simulink model "Vorlage_Gesamtanlage_JaehoCHa"  (R2022a)
settings: Solver=ode3  StartTime=0.0  StopTime=200  FixedStep=0.01  MaxStep=1  MinStep=0.005  RelTol=1e-3  AbsTol=10  EnableMultiTasking=on
values from neighbouring files (symbols this model uses):
  A = 5    [Parameter.m]
  Flaschengroesse = 10    [Parameter.m]
  I = 0.5    [Parameter.m]
  igetr = 1080    [Parameter.m]
  K = 8    [Parameter.m]
  MaxFlaschen = 25    [Parameter.m]
  MRK = 1    [Parameter.m]
  numA = 0    [Parameter.m]
  PassSilo1 = 1    [Parameter.m]
  PassSilo2 = 1    [Parameter.m]
  PHI = 0.001    [Parameter.m]
  Ra = 40    [Parameter.m]
  SizeSilo1 = 15    [Parameter.m]
  SizeSilo2 = 15    [Parameter.m]
  U = 24    [Parameter.m]
  v_band_abfuhr_set = 2    [Parameter.m]
  v_band_arbeit_set = 30    [Parameter.m]
  v_band_zufuhr_set = 10    [Parameter.m]
  v_umsetzer_greifer_set = 400    [Parameter.m]
  v_umsetzer_set = 80    [Parameter.m]
  v_ve1_set = 400    [Parameter.m]
  v_ve2_set = 400    [Parameter.m]
undefined symbols (not defined in the file or in its folder): Limits
libraries: simulink x94
(part 3 of 3)

== system Vorlage_Gesamtanlage_JaehoCHa/Abfüllanlage/Flaschen_data/Flaschenstarter/in_Flaschenzähler ==
  Signal : Inport
  Constant : Constant
  Constant1 : Constant  Value=0
  Logical Operator : Logic  AllPortsSameDT=off
  Memory : Memory
  Memory1 : Memory
  Relational Operator : RelationalOperator  Operator===  InputSameDT=off
  Relational Operator1 : RelationalOperator  Operator===  InputSameDT=off
  Sum : Sum  Inputs=|++  OutDataTypeStr=uint16  SaturateOnIntegerOverflow=on
  Rising Edge : Outport
  Count : Outport  Port=2
  wires:
  Signal/1 -> Memory/1, Relational Operator/2
  Constant/1 -> Relational Operator/1
  Relational Operator/1 -> Logical Operator/1
  Constant1/1 -> Relational Operator1/2
  Memory/1 -> Relational Operator1/1
  Relational Operator1/1 -> Logical Operator/2
  Logical Operator/1 -> Sum/1, Rising Edge/1
  Memory1/1 -> Sum/2
  Sum/1 -> Count/1, Memory1/1

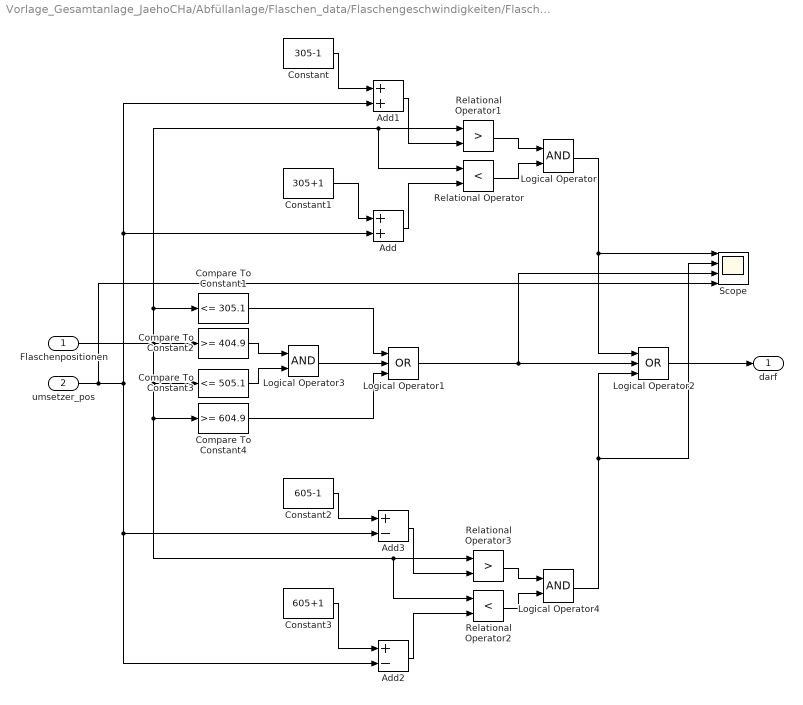
== system Vorlage_Gesamtanlage_JaehoCHa/Abfüllanlage/Flaschen_data/Flaschengeschwindigkeiten/Flaschenabstandsüberwachung/Umsetzer darf mitnehmen ==
  Flaschenpositionen : Inport
  umsetzer_pos : Inport  Port=2
  Add : Sum
  Add1 : Sum
  Add2 : Sum  Inputs=+-
  Add3 : Sum  Inputs=+-
  Compare To Constant1 : simulink/Logic and Bit Operations/Compare To Constant  relop=<=  const=305.1  OutDataTypeStr=uint8  ZeroCross=off
  Compare To Constant2 : simulink/Logic and Bit Operations/Compare To Constant  relop=>=  const=404.9  OutDataTypeStr=uint8  ZeroCross=off
  Compare To Constant3 : simulink/Logic and Bit Operations/Compare To Constant  relop=<=  const=505.1  OutDataTypeStr=uint8  ZeroCross=off
  Compare To Constant4 : simulink/Logic and Bit Operations/Compare To Constant  relop=>=  const=604.9  OutDataTypeStr=uint8  ZeroCross=off
  Constant : Constant  Value=305-1
  Constant1 : Constant  Value=305+1
  Constant2 : Constant  Value=605-1
  Constant3 : Constant  Value=605+1
  Logical Operator : Logic  AllPortsSameDT=off  OutDataTypeStr=boolean
  Logical Operator1 : Logic  Operator=OR  Inputs=3  AllPortsSameDT=off  OutDataTypeStr=boolean
  Logical Operator2 : Logic  Operator=OR  Inputs=3  AllPortsSameDT=off  OutDataTypeStr=boolean
  Logical Operator3 : Logic  AllPortsSameDT=off  OutDataTypeStr=boolean
  Logical Operator4 : Logic  AllPortsSameDT=off  OutDataTypeStr=boolean
  Relational Operator : RelationalOperator  Operator=<  OutDataTypeStr=boolean  InputSameDT=off
  Relational Operator1 : RelationalOperator  Operator=>  OutDataTypeStr=boolean  InputSameDT=off
  Relational Operator2 : RelationalOperator  Operator=<  OutDataTypeStr=boolean  InputSameDT=off
  Relational Operator3 : RelationalOperator  Operator=>  OutDataTypeStr=boolean  InputSameDT=off
  Scope : Scope  NumInputPorts=4
  darf : Outport
  wires:
  Logical Operator2/1 -> darf/1
  Logical Operator1/1 -> Logical Operator2/2, Scope/3
  Compare To Constant1/1 -> Logical Operator1/1
  Logical Operator/1 -> Logical Operator2/1, Scope/1
  Constant/1 -> Add1/1
  Add1/1 -> Relational Operator1/2
  Relational Operator1/1 -> Logical Operator/1
  Relational Operator/1 -> Logical Operator/2
  Add/1 -> Relational Operator/2
  Constant1/1 -> Add/1
  Compare To Constant2/1 -> Logical Operator3/1
  Compare To Constant3/1 -> Logical Operator3/2
  Logical Operator3/1 -> Logical Operator1/2
  Compare To Constant4/1 -> Logical Operator1/3
  Logical Operator4/1 -> Logical Operator2/3, Scope/2
  Constant2/1 -> Add3/1
  Add3/1 -> Relational Operator3/2
  Relational Operator3/1 -> Logical Operator4/1
  Relational Operator2/1 -> Logical Operator4/2
  Add2/1 -> Relational Operator2/2
  Constant3/1 -> Add2/1
  umsetzer_pos/1 -> Add2/2, Add3/2, Add/2, Add1/2, Scope/4
  Flaschenpositionen/1 -> Compare To Constant2/1, Compare To Constant3/1, Compare To Constant4/1, Relational Operator3/1, Relational Operator2/1, Compare To Constant1/1, Relational Operator1/1, Relational Operator/1

== stateflow chart Vorlage_Gesamtanlage_JaehoCHa/Abfüllanlage/Drehscheibe/Sensor ==
  state Start
    en: beep = 0;
  state Beep
    en: beep=1;
  (default) -> Start
  Start -> Beep : [ml.mod(winkel, 90) <=2 | ml.mod(winkel, 90) >=88]
  Beep -> Start : [ml.mod(winkel, 90) >2 && ml.mod(winkel, 90) <88]
  data: winkel input double; beep output boolean

== stateflow chart Vorlage_Gesamtanlage_JaehoCHa/Abfüllanlage/Fehlererkennung/Volle Flasche zum Teller zurück/Chart ==
  state Greife_Flasche_Teller
    entry: error = 0;
  state Oeffne_Greifer_Band
  state Warte_auf_VE2
  state Volle_Flasche_gegriffen
  state Greifer_gestartet
    entry: error = 1;
  state Flasche_weg
  (default) -> Greife_Flasche_Teller
  Flasche_weg -> Greife_Flasche_Teller
  Greife_Flasche_Teller -> Oeffne_Greifer_Band : [I_teller_behaelter_hinten == 1 && i_greifer_zu == 1 && i_umsetz_teller == 1]
  Oeffne_Greifer_Band -> Warte_auf_VE2 : [i_greifer_auf == 1 && i_umsetz_band == 1]
  Volle_Flasche_gegriffen -> Greifer_gestartet [order 1] : [o_umsetz_teller==1]
  Warte_auf_VE2 -> Volle_Flasche_gegriffen [order 2] : [i_greifer_zu == 1]
  Warte_auf_VE2 -> Flasche_weg [order 1] : [i_ve2_herein == 1]
  Volle_Flasche_gegriffen -> Flasche_weg [order 2] : after(5,sec)
  data: I_teller_behaelter_hinten input; i_greifer_zu input; i_umsetz_teller input; i_greifer_auf input; i_umsetz_band input; i_ve2_herein input; error output; o_umsetz_teller input

== stateflow chart Vorlage_Gesamtanlage_JaehoCHa/Steuerung ==
  state Intelligenz [parallel]
    settings: executionOrder=6
    state Anfangszustand
    state Baender_an
      en:send(e_baender_an,Baender);
    state Umsetzer_zu_band
      en:send(e_umsetzer_zu_band,Umsetzer);
      %Bedingung
      %Greifer auf
      %Bedingung nach Fullen
      %Greifer zu
    state Vereinzeler1_open
      en:send(e_ve1_open,VE1_2);
      %Bedingungen
      %Umsetzer auf Band, Greifer ist auf
      %Drehteller ist leer auf der Position
      %keine Flasche an Vereinzeler2
    state Umsetzer_zu_teller
      en:send(e_umsetzer_zu_teller,Umsetzer);
      %Bedingung
      %Greifer zu
    state Greifer_leer_Flasche
      en:send(e_greifer_zu,Umsetzer);
      %Bedingung
      %ve1 offnen
      %eine Flasche an Vereinzeler2
    state Drehteller_ausgerichtet
      en:send(e_Teller_ausgerichtet,Teller);
      %Bedingung
      %Teller ausgerichtet
    state Drehteller_drehen
      en:send(e_Teller_drehen,Teller);
      %Bedingung
      %Greifer open
      % Beidingung nach dem Fulllen
      %warten 2sec
    state Greifer_leer_flasche_los
      en:send(e_greifer_auf,Umsetzer);
      %Bedingung
      %Umsetzer auf Teller
    state Silos_open
      en:send(e_silos_open,Silos);
    state Silos_close
      en:send(e_silos_close,Silos);
    state Greifer_befuellte_Flasche
      en:send(e_greifer_zu,Umsetzer);
    state Umsetzer_zu_band1
      en:send(e_umsetzer_zu_band,Umsetzer);
    state Greifer_befuellte_Flasche_los
      en:send(e_greifer_auf,Umsetzer);
    state Vereinzeler2_open
      en:send(e_ve2_open,VE1_2)
    (default) -> Anfangszustand
    Anfangszustand -> Baender_an
    Baender_an -> Umsetzer_zu_band : [i_umsetzer[3] == 1]
    Greifer_leer_Flasche -> Umsetzer_zu_teller : [i_umsetzer[4] == 1]
    Umsetzer_zu_band -> Vereinzeler1_open : [i_umsetzer[1] == 1 &&i_umsetzer[3]==1&& i_vereinzeler[5] == 1 && i_vereinzeler[6]==0 && i_teller[2]==0]
    Vereinzeler2_open -> Umsetzer_zu_teller [order 2] : [i_silo[2]==1 && i_vereinzeler[5]==0]
    Vereinzeler1_open -> Greifer_leer_Flasche : [ i_vereinzeler[6] == 1]%check
    Silos_close -> Umsetzer_zu_band [order 2] : after(2,sec)[i_teller[2] ==0]%falls keine Flasche auf Teller behaelter
    Drehteller_ausgerichtet -> Umsetzer_zu_band [order 2] : [i_silo[2] == 0 && i_teller[2] ==0]%falls keine Flasche unter Silo und auf Tellerbehaelter
    Umsetzer_zu_teller -> Greifer_leer_flasche_los : [i_umsetzer[2]==1]
    Vereinzeler2_open -> Vereinzeler1_open [order 1] : [i_vereinzeler[4] == 1 && i_vereinzeler[5]==1]%flasche schieben
    Greifer_leer_flasche_los -> Drehteller_drehen : after(2,sec)[i_umsetzer[3]==1]
    Drehteller_drehen -> Drehteller_ausgerichtet : after(0.5,sec)[i_teller[1] == 1]
    Drehteller_ausgerichtet -> Silos_open [order 1] : [i_silo[2]==1 &&(i_silo[3] == 0&&i_silo[4]==0) ] %falls eine Flasche unter teller und beide Silo voll
    Silos_open -> Silos_close : [i_silo[1] == 0]% Flasche unter Silo und voll
    Silos_close -> Greifer_befuellte_Flasche [order 1] : after(2,sec)[i_teller[2]==1]
    Umsetzer_zu_band1 -> Greifer_befuellte_Flasche_los : [i_umsetzer[1]==1]
    Greifer_befuellte_Flasche_los -> Vereinzeler2_open : [i_umsetzer[3]==1&&i_vereinzeler[6]==1]
    Greifer_befuellte_Flasche -> Umsetzer_zu_band1 : [i_umsetzer[4]==1]
  state Umsetzer [parallel]
    settings: executionOrder=1
    state Anfangszustand_Umsetzer
      %umsetzer Band(1), teller(2)
      en:o_umsetzer[1] = 0;
      en:o_umsetzer[2] = 0;
      %Greifer auf(3), zu(4)
      en:o_umsetzer[3] = 1;
      en:o_umsetzer[4] = 0;
      %Umsetzer in Richtung Teller
      %Greifer zu
      %unbenutzte Aktoren soll ausgeschaltet sein.
      %Frage: ist Anfangszustand im Programm schon gegeben ?
    state Bandzustand_Umsetzer
      %umsetzer Band(1), teller(2)
      en:o_umsetzer[1] = 1;
      en:o_umsetzer[2] = 0;
      %Greifer auf(3), zu(4)
      en:o_umsetzer[3] = 0; % schon geoeffnet in Intelligenz
      en:o_umsetzer[4] = 0;
      %Umsetzer wartet auf eine Flasche auf Band
      ex:o_umsetzer[1] =0
    state Bandzustand_Greifer_zu
      %umsetzer Band(1), teller(2)
      en:o_umsetzer[1] = 0;
      en:o_umsetzer[2] = 0;
      %Greifer auf(3), zu(4)
      en:o_umsetzer[3] = 0;
      en:o_umsetzer[4] = 1;
    state Tellerzustand_umsetzer
      %umsetzer Band(1), teller(2)
      en:o_umsetzer[1] = 0;
      en:o_umsetzer[2] = 1;
      %Greifer auf(3), zu(4)
      en:o_umsetzer[3] = 0;
      en:o_umsetzer[4] = 0;
      ex:o_umsetzer[2] = 0;
    state Tellerzustand_Greifer_auf
      %umsetzer Band(1), teller(2)
      en:o_umsetzer[1] = 0;
      en:o_umsetzer[2] = 0;
      %Greifer auf(3), zu(4)
      en:o_umsetzer[3] = 1;
      en:o_umsetzer[4] = 0;
    (default) -> Anfangszustand_Umsetzer
    Bandzustand_Greifer_zu -> Bandzustand_Umsetzer [order 2] : e_umsetzer_zu_band
    Anfangszustand_Umsetzer -> Bandzustand_Umsetzer : e_umsetzer_zu_band
    Tellerzustand_Greifer_auf -> Bandzustand_Greifer_zu [order 1] : e_greifer_zu
    Bandzustand_Umsetzer -> Bandzustand_Greifer_zu [order 1] : e_greifer_zu
    Bandzustand_Greifer_zu -> Tellerzustand_umsetzer [order 1] : e_umsetzer_zu_teller
    Bandzustand_Umsetzer -> Tellerzustand_Greifer_auf [order 2] : e_greifer_auf
    Tellerzustand_Greifer_auf -> Bandzustand_Umsetzer [order 2] : e_umsetzer_zu_band
    Tellerzustand_umsetzer -> Tellerzustand_Greifer_auf : e_greifer_auf
  state Baender [parallel]
    settings: executionOrder=2
    state Arbeitsband_an
      o_band[2] = 1;%arbeitsband eingeschaltet
      %hier muss man korrigieren
    state Anfangszustand_Baender
      o_band[1] = 1; %Zufuhrband eingeschaltet
      o_band[2] = 0; %Arbeitsband ausgeschaltet
    (default) -> Anfangszustand_Baender
    Anfangszustand_Baender -> Arbeitsband_an : e_baender_an[i_band == 1] %i_zufuhr_LT ==1
  state Silos [parallel]
    settings: executionOrder=3
    state Anfangszustand_Soilos
      o_silo[1] = 0;
      o_silo[2] = 0;
    state Anfangszustand_Soilos1
      o_silo[1] = 1;
      o_silo[2] = 1;
    (default) -> Anfangszustand_Soilos
    Anfangszustand_Soilos -> Anfangszustand_Soilos1 : e_silos_open
    Anfangszustand_Soilos1 -> Anfangszustand_Soilos : e_silos_close
  state VE1_2 [parallel]
    settings: executionOrder=4
    state Anfangszustand_vereinzeler
      %Beide Vereinzelergeschlossen
      en:o_vereinzeler[1] =0;
      en:o_vereinzeler[2] =0;
    state open_ve1
      %Vereinzeler 1 wird offen
      en:o_vereinzeler[1] =1;
      en:o_vereinzeler[2] =0;
    state open_ve2
      %Vereinzeler 2 wird offen
      en:o_vereinzeler[1] =0;
      en:o_vereinzeler[2] =1;
    (default) -> Anfangszustand_vereinzeler
    Anfangszustand_vereinzeler -> open_ve1 [order 1] : e_ve1_open
    open_ve1 -> Anfangszustand_vereinzeler : after(1,sec)
    Anfangszustand_vereinzeler -> open_ve2 [order 2] : e_ve2_open
    open_ve2 -> Anfangszustand_vereinzeler : after(1,sec)
  state Teller [parallel]
    settings: executionOrder=5
    state Anfanszustand_teller
      o_teller = 1;
    state Anfanszustand_aus
      o_teller = 0;
    state Anfanszustand_teller_drehen1
      o_teller = 1;
    (default) -> Anfanszustand_teller
    Anfanszustand_teller -> Anfanszustand_aus : [i_teller[1] ==1]
    Anfanszustand_aus -> Anfanszustand_teller_drehen1 : e_Teller_drehen
    Anfanszustand_teller_drehen1 -> Anfanszustand_aus : e_Teller_ausgerichtet
  data: i_band input boolean; o_band output double size=2; o_vereinzeler output double size=2; o_silo output double size=2; o_umsetzer output double size=4; o_teller output double; i_vereinzeler input boolean size=6; i_silo input boolean size=4; i_umsetzer input boolean size=4; i_teller input boolean size=2; clock input double
  events: e_baender_an local FUNCTION_CALL_EVENT; e_umsetzer_zu_band local FUNCTION_CALL_EVENT; e_ve1_open local FUNCTION_CALL_EVENT; e_greifer_zu local FUNCTION_CALL_EVENT; e_umsetzer_zu_teller local FUNCTION_CALL_EVENT; e_Teller_drehen local FUNCTION_CALL_EVENT; e_silos_open local FUNCTION_CALL_EVENT; e_silos_close local FUNCTION_CALL_EVENT; e_Teller_ausgerichtet local FUNCTION_CALL_EVENT; e_greifer_auf local FUNCTION_CALL_EVENT; e_ve2_open local FUNCTION_CALL_EVENT
